simulink model "PROGRAMMING_EXERCISE_PART10"  (R2017b)
settings: Solver=VariableStepAuto  StartTime=0.0  StopTime=3  RelTol=1e-3
settings Model: Creator=chenjiasheng  LastModifiedBy=chenjiasheng

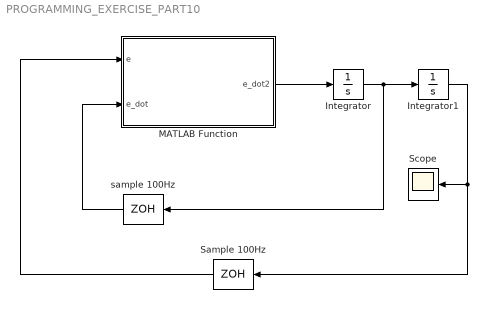
== system PROGRAMMING_EXERCISE_PART10 ==
  Integrator : Integrator  InitialCondition=[0 0 0]'
  Integrator1 : Integrator  InitialCondition=[0 60 0]'
  MATLAB Function : MATLAB Function  TreatAsAtomicUnit=on
  Sample 100Hz : ZeroOrderHold  SampleTime=0.01
  Scope : Scope
  sample 100Hz : ZeroOrderHold  SampleTime=0.01
  wires:
  MATLAB Function/1(e_dot2) -> Integrator/1
  Integrator/1 -> sample 100Hz/1, Integrator1/1
  Integrator1/1 -> Scope/1, Sample 100Hz/1
  Sample 100Hz/1 -> MATLAB Function/1(e)
  sample 100Hz/1 -> MATLAB Function/2(e_dot)

== matlab function PROGRAMMING_EXERCISE_PART10/MATLAB Function ==
  data: e input; e_dot2 output; e_dot input
function e_dot2 = fcn(e,e_dot)
e_dot2=-[100 0   0;
         0   100 0;
         0   0   100]*e-[20 0  0;
                         0  20 0;
                         0  0  20]*e_dot;
end
